simulink model "HBsimDC"  (R2018b)
settings: Solver=ode4  StartTime=0.0  StopTime=0.5e-3*1+0.05*2*0  FixedStep=Tsim  MaxStep=1e-4  RelTol=1e-6
undefined symbols (not defined in the file): fsw, J, Kt, La, Ra, sigbuilder_block, Vdc
libraries: powerlib x7, simulink x2, powerlib_meascontrol x1
settings Model: Creator=matti  LastModifiedBy=matti
settings DataIOCC: ReturnWorkspaceOutputs=on

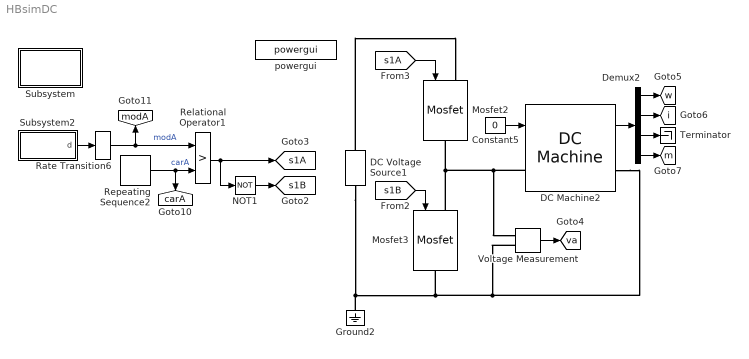
== system HBsimDC ==
  Constant5 : Constant  Value=0  SampleTime=1/(200*fsw)
  DC Machine2 : powerlib/Machines/DC Machine  PresetModel=No  MechanicalLoad=Torque TL  FieldType=Permanent magnet  ShowDetailedParameters=on  MeasurementBus=off  RLa="[Ra  La]"  RLf="[ 240  120]"  Laf=1.8  MachineConstant=Torque constant (N.m/A)  Ke=1.8  Kt=Kt  J=J  Bm=B  Tf=0  w0=0  Ifinit=1  TsPowergui=0  TsBlock=-1
      settings: SourceProductName=Simscape Electrical
  DC Voltage Source1 : powerlib/Electrical Sources/DC Voltage Source  Amplitude=Vdc  Measurements=None
      settings: SourceProductName=Simscape Electrical
  Demux2 : Demux  BusSelectionMode=on
  Ground2 : powerlib/Elements/Ground  LConnTagsString=a
      settings: SourceProductName=Simscape Electrical
  Mosfet2 : powerlib/Power Electronics/Mosfet  Ron=0.1  Lon=0  Rd=0.01  Vfd=0  IC=0  Rs=1e5  Cs=inf  Measurements=off
      settings: SourceProductName=Simscape Electrical
  Mosfet3 : powerlib/Power Electronics/Mosfet  Ron=0.1  Lon=0  Rd=0.01  Vfd=0  IC=0  Rs=1e5  Cs=inf  Measurements=off
      settings: SourceProductName=Simscape Electrical
  NOT1 : Logic  Operator=NOT  IconShape=distinctive  AllPortsSameDT=off  OutDataTypeStr=boolean
  Rate Transition6 : RateTransition  OutPortSampleTime=Ts
  Relational Operator1 : RelationalOperator  Operator=>  OutDataTypeStr=boolean  RndMeth=Simplest
  Repeating Sequence2 : simulink/Sources/Repeating Sequence  rep_seq_t=[0 1/(2*fsw) 1/fsw]  rep_seq_y=[0 1 0]
  Subsystem : Subsystem
      mask Display: disp('stream')
  Subsystem2 : Subsystem
      mask Display: disp('reference')
  Terminator : Terminator
  Voltage Measurement : powerlib/Measurements/Voltage Measurement  PhasorSimulation=off  OutputType=Complex  PSBequivalent=0
      settings: SourceProductName=Simscape Electrical
  powergui : powerlib/powergui  Priority=1  SimulationMode=Continuous  SampleTime=1/(400*fsw)  frequency=60  Iterations=50  frequencyindice=0  Pbase=100e6  ErrMax=1e-4  UnitsV=kV  UnitsW=MW  buscounter=0  FunctionMessages=off  echomessages=off  EnableUseOfTLC=off  CurrentSourceSwitches=off  DisableSnubberDevices=on  DisableRonSwitches=on  DisableVfSwitches=on  DisplayEquations=off  SolverType=Tustin/Backward Euler (TBE)  Interpol=off  ExternalGateDelay=off  methode=off  Ts=100  x0status=blocks  SPID=off  SwTol=0  HookPort=off  RestoreLinks=warning  ResistiveCurrentMeasurement=off  Frange=[0:2:500]  Ylog=off  Xlog=on  ShowGrid=off  save=off  variable=ZData  structure=0  ZoomFFT=off  StartTime=0.0  cycles=1  DisplayStyle=1  fundamental=60  FreqAxis=off  MaxFrequency=1000  frequencyindicesteady=1  RmsSteady=1  display=off
  tag scope: carA=global, i=global, m=global, modA=global, s1A=global, s1B=global, va=global, w=global
  wires:
  Relational Operator1/1 -> NOT1/1, [s1A]
  NOT1/1 -> [s1B]
  DC Machine2/1 -> Demux2/1
  [s1B] -> Mosfet3/1
  [s1A] -> Mosfet2/1
  Demux2/3 -> Terminator/1
  Voltage Measurement/1 -> [va]
  Repeating Sequence2/1 -> [carA], Relational Operator1/2  "carA"
  Subsystem2/1(d) -> Rate Transition6/1
  Constant5/1 -> DC Machine2/1
  Demux2/1 -> [w]
  Demux2/2 -> [i]
  Demux2/4 -> [m]
  Rate Transition6/1 -> Relational Operator1/1, [modA]  "modA"
  connections:
  Ground2/LConn1 -- DC Voltage Source1/LConn1 -- Voltage Measurement/LConn2 -- DC Machine2/RConn1 -- Mosfet3/RConn1
  DC Voltage Source1/RConn1 -- Mosfet2/LConn1
  Mosfet3/LConn1 -- DC Machine2/LConn1 -- Voltage Measurement/LConn1 -- Mosfet2/RConn1

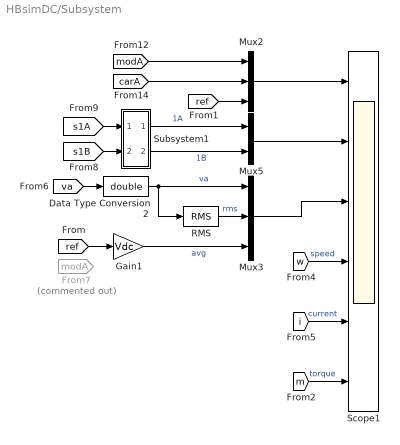
== system HBsimDC/Subsystem ==
  Data Type Conversion2 : DataTypeConversion  OutDataTypeStr=double
  From7 : From  Commented=on  GotoTag=modA  TagVisibility=global
  Gain1 : Gain  Gain=Vdc
  Mux2 : Mux  Inputs=3
  Mux3 : Mux  Inputs=3
  Mux5 : Mux  Inputs=2
  RMS : powerlib_meascontrol/Measurements/RMS  TrueRMS=on  Freq=fsw  RMSInit=0  Ts=0
  Scope1 : Scope  NumInputPorts=6
  Subsystem1 : Subsystem
      mask Display: disp('shift')
  wires:
  [ref] -> Gain1/1
  [modA] -> Mux2/1
  Mux3/1 -> Scope1/3
  [carA] -> Mux2/2
  [s1A] -> Subsystem1/1(In1)
  Gain1/1 -> Mux3/3  "avg"
  [va] -> Data Type Conversion2/1
  Data Type Conversion2/1 -> RMS/1, Mux3/1  "va"
  [s1B] -> Subsystem1/2(In2)
  Subsystem1/2(Out2) -> Mux5/2  "1B"
  Subsystem1/1(Out1) -> Mux5/1  "1A"
  Mux5/1 -> Scope1/2
  [w] -> Scope1/4  "speed"
  [i] -> Scope1/5  "current"
  [m] -> Scope1/6  "torque"
  Mux2/1 -> Scope1/1
  [ref] -> Mux2/3
  RMS/1 -> Mux3/2  "rms"

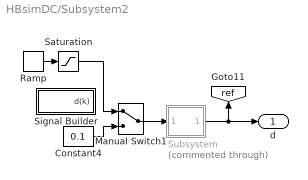
== system HBsimDC/Subsystem2 ==
  Constant4 : Constant  Value=0.1  SampleTime=1/(200*fsw)
  Manual Switch1 : ManualSwitch
  Ramp : simulink/Sources/Ramp  slope=0.9/3e-4  start=0  InitialOutput=0
  Saturation : Saturate  UpperLimit=0.9  LowerLimit=0
  Signal Builder : Subsystem  Tag=STV Subsys  LoadFcn=sigbuilder_block('load');  StartFcn=sigbuilder_block('start');  StopFcn=sigbuilder_block('stop');  ClipboardFcn=sigbuilder_block('clipboard');  mask(Sigbuilder block){tuvar=[0:10]}
      mask help: Simulink:masks:SigbuilderBlock_MD
      mask init:
      | if ~strcmp(get_param(bdroot(gcbh),'SimulationStatus'),'stopped') tuvar = sigbuilder_block('maskInit'); end
      settings: CopyFcn=sigbuilder_block('copy');  DeleteFcn=sigbuilder_block('delete');  ModelCloseFcn=sigbuilder_block('modelClose');  PreSaveFcn=sigbuilder_block('preSave');  PauseFcn=sigbuilder_block('pause');  ContinueFcn=sigbuilder_block('continue');  NameChangeFcn=sigbuilder_block('namechange');  OpenFcn=sigbuilder_block('open',[437.6 199.2 550.4 400 ]);  CloseFcn=sigbuilder_block('close');
      mask Display: plot(0, 0, 100, 100,[2, 2, 32, 32, 2], [68, 8, 8, 68, 68],[32, 2], [38, 38], [32, 19, 2],[53, 60, 44], [32, 17, 17, 2],[16, 16, 31, 31]);txt = getActiveGroup(gcbh);text(2, 100, txt,'verticalAlignment', 'top');
  Subsystem : Subsystem  Commented=through
      mask Display: disp('cut\nnoise')
  d : Outport
  tag scope: ref=global
  wires:
  Saturation/1 -> Manual Switch1/1
  Constant4/1 -> Manual Switch1/2
  Manual Switch1/1 -> Subsystem/1(In1)
  Subsystem/1(Out1) -> [ref], d/1
  Ramp/1 -> Saturation/1

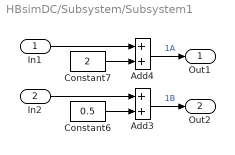
== system HBsimDC/Subsystem/Subsystem1 ==
  In1 : Inport
  In2 : Inport  Port=2
  Add3 : Sum
  Add4 : Sum
  Constant6 : Constant  Value=0.5  SampleTime=1/(200*fsw)
  Constant7 : Constant  Value=2  SampleTime=1/(200*fsw)
  Out1 : Outport
  Out2 : Outport  Port=2
  wires:
  In2/1 -> Add3/1
  In1/1 -> Add4/1
  Constant6/1 -> Add3/2
  Constant7/1 -> Add4/2
  Add4/1 -> Out1/1  "1A"
  Add3/1 -> Out2/1  "1B"

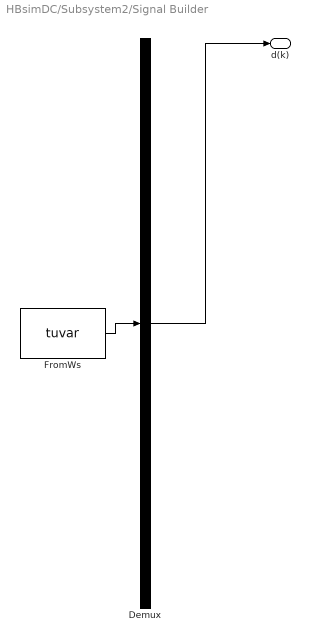
== system HBsimDC/Subsystem2/Signal Builder ==
  Demux : Demux  Tag=STV Demux  Outputs=1
  FromWs : FromWorkspace  Tag=STV FromWs  VariableName=tuvar  SampleTime=0
      SigBuilderData=|
      | common.afterFinalStr = 'Extrapolate'
      | common.sampleTime = 0
      | dataSet.timeRange = [0 0.12]
      | dataSet.name = '  '
      | sbobj.Groups.Name = '  '
      | sbobj.Groups.Signals.Name = 'd(k)'
      | sbobj.Groups.Signals.XData = [0 0.015 0.05 0.06 0.1 0.11 0.12]
      | sbobj.Groups.Signals.YData = [0.05 0.9 0.9 0.6 0.6 0 0]
      | sbobj.Groups.TimeRange = [0 0.12]
  d(k) : Outport  Tag=STV Outport
  wires:
  Demux/1 -> d(k)/1
  FromWs/1 -> Demux/1

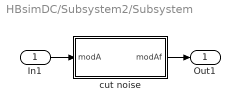
== system HBsimDC/Subsystem2/Subsystem ==
  In1 : Inport
  cut noise : MATLAB Function  TreatAsAtomicUnit=on
  Out1 : Outport
  wires:
  In1/1 -> cut noise/1(modA)
  cut noise/1(modAf) -> Out1/1

== matlab function HBsimDC/Subsystem2/Subsystem/cut noise ==
  data: modA input; modAf output
function modAf = cutter(modA)
if modA <= 0.5002 && modA >= 0.4998
    modAf = 0.5;
else
    modAf = modA;
end
